simulink model "signal_tranmission"  (R2024b)
settings: Solver=ode45  StartTime=0.0  StopTime=10  FixedStep=0.000125  RelTol=1e-3
libraries: dspfdesign x500, commchan3 x1
(part 4 of 7)

== system signal_tranmission/SSB Modulator85 ==
  Input Signal : Inport
  Analog Filter Design : dspfdesign/Analog Filter Design  method=Butterworth  filttype=Bandpass  N=4  Wlo=438*2*pi  Whi=442*2*pi  Rp=2  Rs=40
  Balanced Modulator : Subsystem
  carrier signal : Sin  Frequency=440*2*pi  SampleTime=0
  Out1 : Outport
  wires:
  carrier signal/1 -> Balanced Modulator/2(Carrier Signal)
  Balanced Modulator/1(DSBSC) -> Analog Filter Design/1
  Analog Filter Design/1 -> Out1/1
  Input Signal/1 -> Balanced Modulator/1(Input Signal)

== system signal_tranmission/SSB Modulator86 ==
  Input Signal : Inport
  Analog Filter Design : dspfdesign/Analog Filter Design  method=Butterworth  filttype=Bandpass  N=4  Wlo=442*2*pi  Whi=446*2*pi  Rp=2  Rs=40
  Balanced Modulator : Subsystem
  carrier signal : Sin  Frequency=444*2*pi  SampleTime=0
  Out1 : Outport
  wires:
  carrier signal/1 -> Balanced Modulator/2(Carrier Signal)
  Balanced Modulator/1(DSBSC) -> Analog Filter Design/1
  Analog Filter Design/1 -> Out1/1
  Input Signal/1 -> Balanced Modulator/1(Input Signal)

== system signal_tranmission/SSB Modulator87 ==
  Input Signal : Inport
  Analog Filter Design : dspfdesign/Analog Filter Design  method=Butterworth  filttype=Bandpass  N=4  Wlo=446*2*pi  Whi=450*2*pi  Rp=2  Rs=40
  Balanced Modulator : Subsystem
  carrier signal : Sin  Frequency=448*2*pi  SampleTime=0
  Out1 : Outport
  wires:
  carrier signal/1 -> Balanced Modulator/2(Carrier Signal)
  Balanced Modulator/1(DSBSC) -> Analog Filter Design/1
  Analog Filter Design/1 -> Out1/1
  Input Signal/1 -> Balanced Modulator/1(Input Signal)

== system signal_tranmission/SSB Modulator88 ==
  Input Signal : Inport
  Analog Filter Design : dspfdesign/Analog Filter Design  method=Butterworth  filttype=Bandpass  N=4  Wlo=450*2*pi  Whi=454*2*pi  Rp=2  Rs=40
  Balanced Modulator : Subsystem
  carrier signal : Sin  Frequency=452*2*pi  SampleTime=0
  Out1 : Outport
  wires:
  carrier signal/1 -> Balanced Modulator/2(Carrier Signal)
  Balanced Modulator/1(DSBSC) -> Analog Filter Design/1
  Analog Filter Design/1 -> Out1/1
  Input Signal/1 -> Balanced Modulator/1(Input Signal)

== system signal_tranmission/SSB Modulator89 ==
  Input Signal : Inport
  Analog Filter Design : dspfdesign/Analog Filter Design  method=Butterworth  filttype=Bandpass  N=4  Wlo=454*2*pi  Whi=458*2*pi  Rp=2  Rs=40
  Balanced Modulator : Subsystem
  carrier signal : Sin  Frequency=456*2*pi  SampleTime=0
  Out1 : Outport
  wires:
  carrier signal/1 -> Balanced Modulator/2(Carrier Signal)
  Balanced Modulator/1(DSBSC) -> Analog Filter Design/1
  Analog Filter Design/1 -> Out1/1
  Input Signal/1 -> Balanced Modulator/1(Input Signal)

== system signal_tranmission/SSB Modulator9 ==
  Input Signal : Inport
  Analog Filter Design : dspfdesign/Analog Filter Design  method=Butterworth  filttype=Bandpass  N=4  Wlo=134*2*pi  Whi=138*2*pi  Rp=2  Rs=40
  Balanced Modulator : Subsystem
  carrier signal : Sin  Frequency=136*2*pi  SampleTime=0
  Out1 : Outport
  wires:
  carrier signal/1 -> Balanced Modulator/2(Carrier Signal)
  Balanced Modulator/1(DSBSC) -> Analog Filter Design/1
  Analog Filter Design/1 -> Out1/1
  Input Signal/1 -> Balanced Modulator/1(Input Signal)

== system signal_tranmission/SSB Modulator90 ==
  Input Signal : Inport
  Analog Filter Design : dspfdesign/Analog Filter Design  method=Butterworth  filttype=Bandpass  N=4  Wlo=458*2*pi  Whi=462*2*pi  Rp=2  Rs=40
  Balanced Modulator : Subsystem
  carrier signal : Sin  Frequency=460*2*pi  SampleTime=0
  Out1 : Outport
  wires:
  carrier signal/1 -> Balanced Modulator/2(Carrier Signal)
  Balanced Modulator/1(DSBSC) -> Analog Filter Design/1
  Analog Filter Design/1 -> Out1/1
  Input Signal/1 -> Balanced Modulator/1(Input Signal)

== system signal_tranmission/SSB Modulator91 ==
  Input Signal : Inport
  Analog Filter Design : dspfdesign/Analog Filter Design  method=Butterworth  filttype=Bandpass  N=4  Wlo=462*2*pi  Whi=466*2*pi  Rp=2  Rs=40
  Balanced Modulator : Subsystem
  carrier signal : Sin  Frequency=464*2*pi  SampleTime=0
  Out1 : Outport
  wires:
  carrier signal/1 -> Balanced Modulator/2(Carrier Signal)
  Balanced Modulator/1(DSBSC) -> Analog Filter Design/1
  Analog Filter Design/1 -> Out1/1
  Input Signal/1 -> Balanced Modulator/1(Input Signal)

== system signal_tranmission/SSB Modulator92 ==
  Input Signal : Inport
  Analog Filter Design : dspfdesign/Analog Filter Design  method=Butterworth  filttype=Bandpass  N=4  Wlo=466*2*pi  Whi=470*2*pi  Rp=2  Rs=40
  Balanced Modulator : Subsystem
  carrier signal : Sin  Frequency=468*2*pi  SampleTime=0
  Out1 : Outport
  wires:
  carrier signal/1 -> Balanced Modulator/2(Carrier Signal)
  Balanced Modulator/1(DSBSC) -> Analog Filter Design/1
  Analog Filter Design/1 -> Out1/1
  Input Signal/1 -> Balanced Modulator/1(Input Signal)

== system signal_tranmission/SSB Modulator93 ==
  Input Signal : Inport
  Analog Filter Design : dspfdesign/Analog Filter Design  method=Butterworth  filttype=Bandpass  N=4  Wlo=470*2*pi  Whi=474*2*pi  Rp=2  Rs=40
  Balanced Modulator : Subsystem
  carrier signal : Sin  Frequency=472*2*pi  SampleTime=0
  Out1 : Outport
  wires:
  carrier signal/1 -> Balanced Modulator/2(Carrier Signal)
  Balanced Modulator/1(DSBSC) -> Analog Filter Design/1
  Analog Filter Design/1 -> Out1/1
  Input Signal/1 -> Balanced Modulator/1(Input Signal)

== system signal_tranmission/SSB Modulator94 ==
  Input Signal : Inport
  Analog Filter Design : dspfdesign/Analog Filter Design  method=Butterworth  filttype=Bandpass  N=4  Wlo=474*2*pi  Whi=478*2*pi  Rp=2  Rs=40
  Balanced Modulator : Subsystem
  carrier signal : Sin  Frequency=476*2*pi  SampleTime=0
  Out1 : Outport
  wires:
  carrier signal/1 -> Balanced Modulator/2(Carrier Signal)
  Balanced Modulator/1(DSBSC) -> Analog Filter Design/1
  Analog Filter Design/1 -> Out1/1
  Input Signal/1 -> Balanced Modulator/1(Input Signal)

== system signal_tranmission/SSB Modulator95 ==
  Input Signal : Inport
  Analog Filter Design : dspfdesign/Analog Filter Design  method=Butterworth  filttype=Bandpass  N=4  Wlo=478*2*pi  Whi=482*2*pi  Rp=2  Rs=40
  Balanced Modulator : Subsystem
  carrier signal : Sin  Frequency=480*2*pi  SampleTime=0
  Out1 : Outport
  wires:
  carrier signal/1 -> Balanced Modulator/2(Carrier Signal)
  Balanced Modulator/1(DSBSC) -> Analog Filter Design/1
  Analog Filter Design/1 -> Out1/1
  Input Signal/1 -> Balanced Modulator/1(Input Signal)

== system signal_tranmission/SSB Modulator96 ==
  Input Signal : Inport
  Analog Filter Design : dspfdesign/Analog Filter Design  method=Butterworth  filttype=Bandpass  N=4  Wlo=482*2*pi  Whi=486*2*pi  Rp=2  Rs=40
  Balanced Modulator : Subsystem
  carrier signal : Sin  Frequency=484*2*pi  SampleTime=0
  Out1 : Outport
  wires:
  carrier signal/1 -> Balanced Modulator/2(Carrier Signal)
  Balanced Modulator/1(DSBSC) -> Analog Filter Design/1
  Analog Filter Design/1 -> Out1/1
  Input Signal/1 -> Balanced Modulator/1(Input Signal)

== system signal_tranmission/SSB Modulator97 ==
  Input Signal : Inport
  Analog Filter Design : dspfdesign/Analog Filter Design  method=Butterworth  filttype=Bandpass  N=4  Wlo=486*2*pi  Whi=490*2*pi  Rp=2  Rs=40
  Balanced Modulator : Subsystem
  carrier signal : Sin  Frequency=488*2*pi  SampleTime=0
  Out1 : Outport
  wires:
  carrier signal/1 -> Balanced Modulator/2(Carrier Signal)
  Balanced Modulator/1(DSBSC) -> Analog Filter Design/1
  Analog Filter Design/1 -> Out1/1
  Input Signal/1 -> Balanced Modulator/1(Input Signal)

== system signal_tranmission/SSB Modulator98 ==
  Input Signal : Inport
  Analog Filter Design : dspfdesign/Analog Filter Design  method=Butterworth  filttype=Bandpass  N=4  Wlo=490*2*pi  Whi=494*2*pi  Rp=2  Rs=40
  Balanced Modulator : Subsystem
  carrier signal : Sin  Frequency=492*2*pi  SampleTime=0
  Out1 : Outport
  wires:
  carrier signal/1 -> Balanced Modulator/2(Carrier Signal)
  Balanced Modulator/1(DSBSC) -> Analog Filter Design/1
  Analog Filter Design/1 -> Out1/1
  Input Signal/1 -> Balanced Modulator/1(Input Signal)

== system signal_tranmission/SSB Modulator99 ==
  Input Signal : Inport
  Analog Filter Design : dspfdesign/Analog Filter Design  method=Butterworth  filttype=Bandpass  N=4  Wlo=494*2*pi  Whi=498*2*pi  Rp=2  Rs=40
  Balanced Modulator : Subsystem
  carrier signal : Sin  Frequency=496*2*pi  SampleTime=0
  Out1 : Outport
  wires:
  carrier signal/1 -> Balanced Modulator/2(Carrier Signal)
  Balanced Modulator/1(DSBSC) -> Analog Filter Design/1
  Analog Filter Design/1 -> Out1/1
  Input Signal/1 -> Balanced Modulator/1(Input Signal)

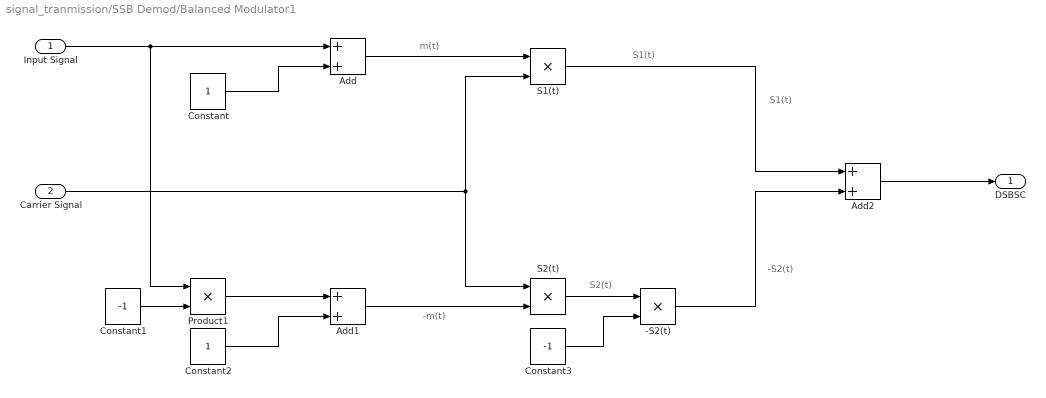
== system signal_tranmission/SSB Demod/Balanced Modulator1 ==
  note: -S2(t)
  note: S1(t)
  note: -m(t)
  note: m(t)
  note: S2(t)
  note: S1(t)
  Input Signal : Inport
  Carrier Signal : Inport  Port=2
  -S2(t) : Product
  Add : Sum
  Add1 : Sum
  Add2 : Sum
  Constant : Constant
  Constant1 : Constant  Value=-1
  Constant2 : Constant
  Constant3 : Constant  Value=-1
  Product1 : Product
  S1(t) : Product
  S2(t) : Product
  DSBSC : Outport
  wires:
  Product1/1 -> Add1/1
  Add/1 -> S1(t)/1
  Constant3/1 -> -S2(t)/2
  Constant2/1 -> Add1/2
  S2(t)/1 -> -S2(t)/1
  Carrier Signal/1 -> S1(t)/2, S2(t)/1
  Constant/1 -> Add/2
  Add1/1 -> S2(t)/2
  Constant1/1 -> Product1/2
  -S2(t)/1 -> Add2/2
  S1(t)/1 -> Add2/1
  Input Signal/1 -> Product1/1, Add/1
  Add2/1 -> DSBSC/1

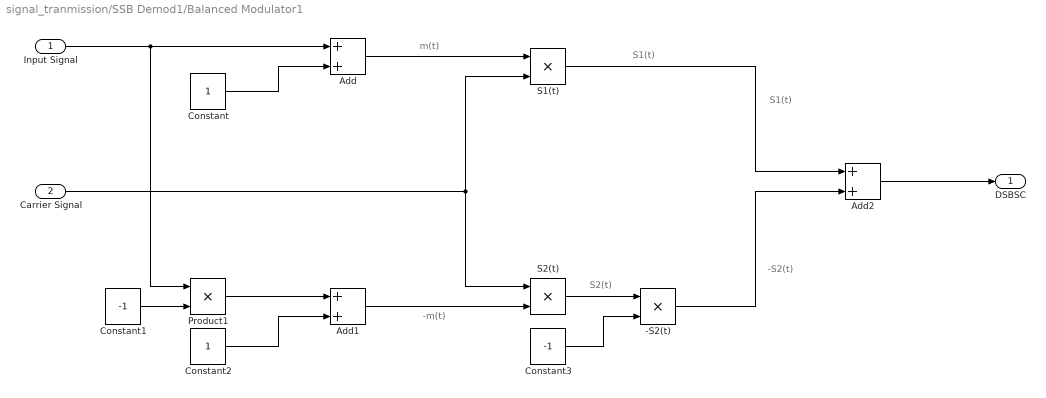
== system signal_tranmission/SSB Demod1/Balanced Modulator1 ==
  note: -S2(t)
  note: S1(t)
  note: -m(t)
  note: m(t)
  note: S2(t)
  note: S1(t)
  Input Signal : Inport
  Carrier Signal : Inport  Port=2
  -S2(t) : Product
  Add : Sum
  Add1 : Sum
  Add2 : Sum
  Constant : Constant
  Constant1 : Constant  Value=-1
  Constant2 : Constant
  Constant3 : Constant  Value=-1
  Product1 : Product
  S1(t) : Product
  S2(t) : Product
  DSBSC : Outport
  wires:
  Product1/1 -> Add1/1
  Add/1 -> S1(t)/1
  Constant3/1 -> -S2(t)/2
  Constant2/1 -> Add1/2
  S2(t)/1 -> -S2(t)/1
  Carrier Signal/1 -> S1(t)/2, S2(t)/1
  Constant/1 -> Add/2
  Add1/1 -> S2(t)/2
  Constant1/1 -> Product1/2
  -S2(t)/1 -> Add2/2
  S1(t)/1 -> Add2/1
  Input Signal/1 -> Product1/1, Add/1
  Add2/1 -> DSBSC/1

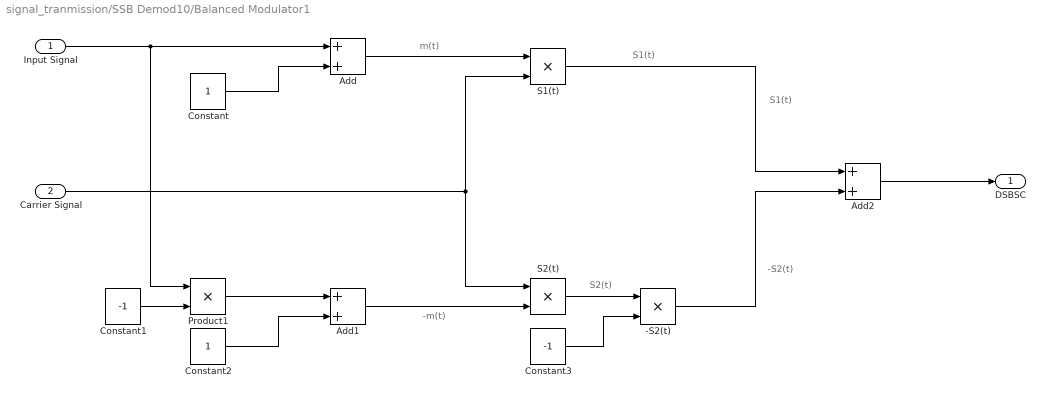
== system signal_tranmission/SSB Demod10/Balanced Modulator1 ==
  note: -S2(t)
  note: S1(t)
  note: -m(t)
  note: m(t)
  note: S2(t)
  note: S1(t)
  Input Signal : Inport
  Carrier Signal : Inport  Port=2
  -S2(t) : Product
  Add : Sum
  Add1 : Sum
  Add2 : Sum
  Constant : Constant
  Constant1 : Constant  Value=-1
  Constant2 : Constant
  Constant3 : Constant  Value=-1
  Product1 : Product
  S1(t) : Product
  S2(t) : Product
  DSBSC : Outport
  wires:
  Product1/1 -> Add1/1
  Add/1 -> S1(t)/1
  Constant3/1 -> -S2(t)/2
  Constant2/1 -> Add1/2
  S2(t)/1 -> -S2(t)/1
  Carrier Signal/1 -> S1(t)/2, S2(t)/1
  Constant/1 -> Add/2
  Add1/1 -> S2(t)/2
  Constant1/1 -> Product1/2
  -S2(t)/1 -> Add2/2
  S1(t)/1 -> Add2/1
  Input Signal/1 -> Product1/1, Add/1
  Add2/1 -> DSBSC/1

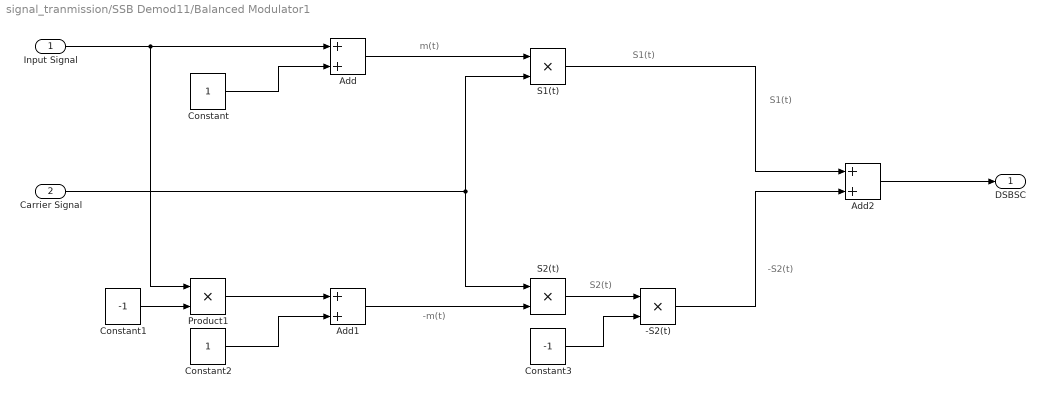
== system signal_tranmission/SSB Demod11/Balanced Modulator1 ==
  note: -S2(t)
  note: S1(t)
  note: -m(t)
  note: m(t)
  note: S2(t)
  note: S1(t)
  Input Signal : Inport
  Carrier Signal : Inport  Port=2
  -S2(t) : Product
  Add : Sum
  Add1 : Sum
  Add2 : Sum
  Constant : Constant
  Constant1 : Constant  Value=-1
  Constant2 : Constant
  Constant3 : Constant  Value=-1
  Product1 : Product
  S1(t) : Product
  S2(t) : Product
  DSBSC : Outport
  wires:
  Product1/1 -> Add1/1
  Add/1 -> S1(t)/1
  Constant3/1 -> -S2(t)/2
  Constant2/1 -> Add1/2
  S2(t)/1 -> -S2(t)/1
  Carrier Signal/1 -> S1(t)/2, S2(t)/1
  Constant/1 -> Add/2
  Add1/1 -> S2(t)/2
  Constant1/1 -> Product1/2
  -S2(t)/1 -> Add2/2
  S1(t)/1 -> Add2/1
  Input Signal/1 -> Product1/1, Add/1
  Add2/1 -> DSBSC/1

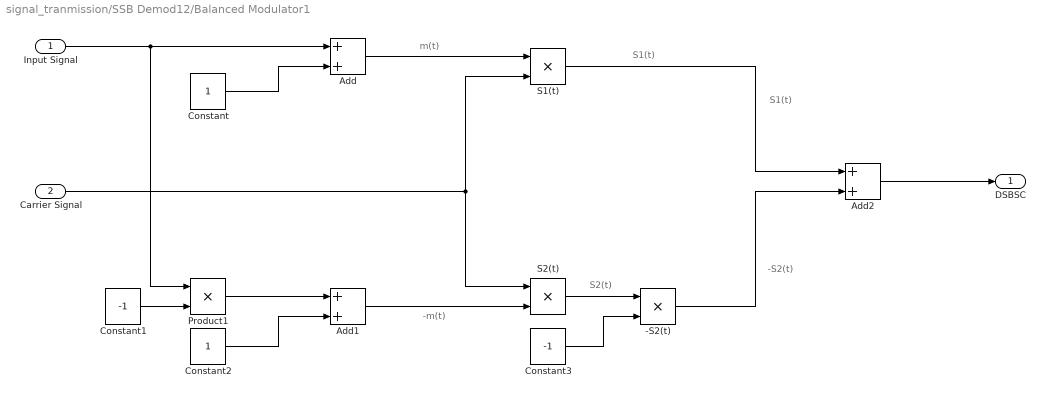
== system signal_tranmission/SSB Demod12/Balanced Modulator1 ==
  note: -S2(t)
  note: S1(t)
  note: -m(t)
  note: m(t)
  note: S2(t)
  note: S1(t)
  Input Signal : Inport
  Carrier Signal : Inport  Port=2
  -S2(t) : Product
  Add : Sum
  Add1 : Sum
  Add2 : Sum
  Constant : Constant
  Constant1 : Constant  Value=-1
  Constant2 : Constant
  Constant3 : Constant  Value=-1
  Product1 : Product
  S1(t) : Product
  S2(t) : Product
  DSBSC : Outport
  wires:
  Product1/1 -> Add1/1
  Add/1 -> S1(t)/1
  Constant3/1 -> -S2(t)/2
  Constant2/1 -> Add1/2
  S2(t)/1 -> -S2(t)/1
  Carrier Signal/1 -> S1(t)/2, S2(t)/1
  Constant/1 -> Add/2
  Add1/1 -> S2(t)/2
  Constant1/1 -> Product1/2
  -S2(t)/1 -> Add2/2
  S1(t)/1 -> Add2/1
  Input Signal/1 -> Product1/1, Add/1
  Add2/1 -> DSBSC/1

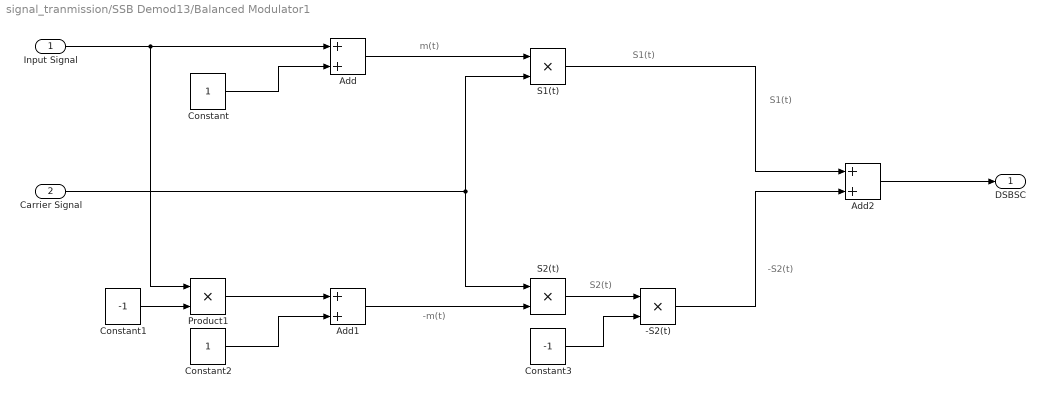
== system signal_tranmission/SSB Demod13/Balanced Modulator1 ==
  note: -S2(t)
  note: S1(t)
  note: -m(t)
  note: m(t)
  note: S2(t)
  note: S1(t)
  Input Signal : Inport
  Carrier Signal : Inport  Port=2
  -S2(t) : Product
  Add : Sum
  Add1 : Sum
  Add2 : Sum
  Constant : Constant
  Constant1 : Constant  Value=-1
  Constant2 : Constant
  Constant3 : Constant  Value=-1
  Product1 : Product
  S1(t) : Product
  S2(t) : Product
  DSBSC : Outport
  wires:
  Product1/1 -> Add1/1
  Add/1 -> S1(t)/1
  Constant3/1 -> -S2(t)/2
  Constant2/1 -> Add1/2
  S2(t)/1 -> -S2(t)/1
  Carrier Signal/1 -> S1(t)/2, S2(t)/1
  Constant/1 -> Add/2
  Add1/1 -> S2(t)/2
  Constant1/1 -> Product1/2
  -S2(t)/1 -> Add2/2
  S1(t)/1 -> Add2/1
  Input Signal/1 -> Product1/1, Add/1
  Add2/1 -> DSBSC/1

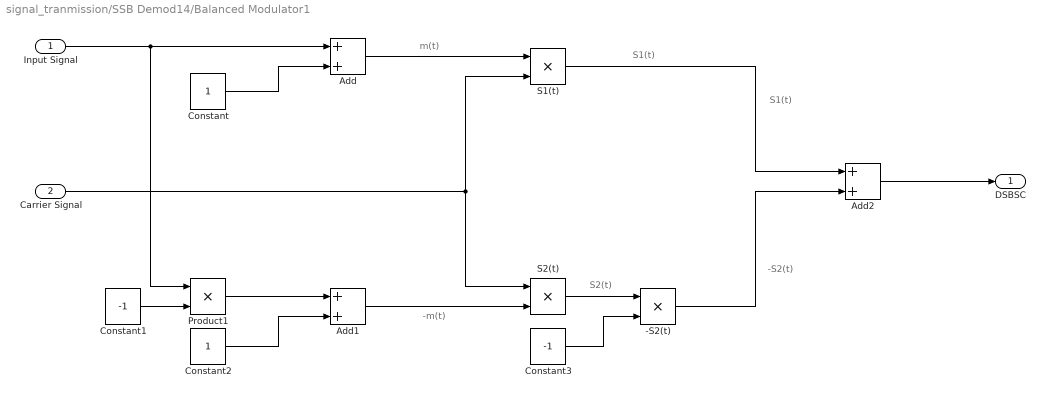
== system signal_tranmission/SSB Demod14/Balanced Modulator1 ==
  note: -S2(t)
  note: S1(t)
  note: -m(t)
  note: m(t)
  note: S2(t)
  note: S1(t)
  Input Signal : Inport
  Carrier Signal : Inport  Port=2
  -S2(t) : Product
  Add : Sum
  Add1 : Sum
  Add2 : Sum
  Constant : Constant
  Constant1 : Constant  Value=-1
  Constant2 : Constant
  Constant3 : Constant  Value=-1
  Product1 : Product
  S1(t) : Product
  S2(t) : Product
  DSBSC : Outport
  wires:
  Product1/1 -> Add1/1
  Add/1 -> S1(t)/1
  Constant3/1 -> -S2(t)/2
  Constant2/1 -> Add1/2
  S2(t)/1 -> -S2(t)/1
  Carrier Signal/1 -> S1(t)/2, S2(t)/1
  Constant/1 -> Add/2
  Add1/1 -> S2(t)/2
  Constant1/1 -> Product1/2
  -S2(t)/1 -> Add2/2
  S1(t)/1 -> Add2/1
  Input Signal/1 -> Product1/1, Add/1
  Add2/1 -> DSBSC/1

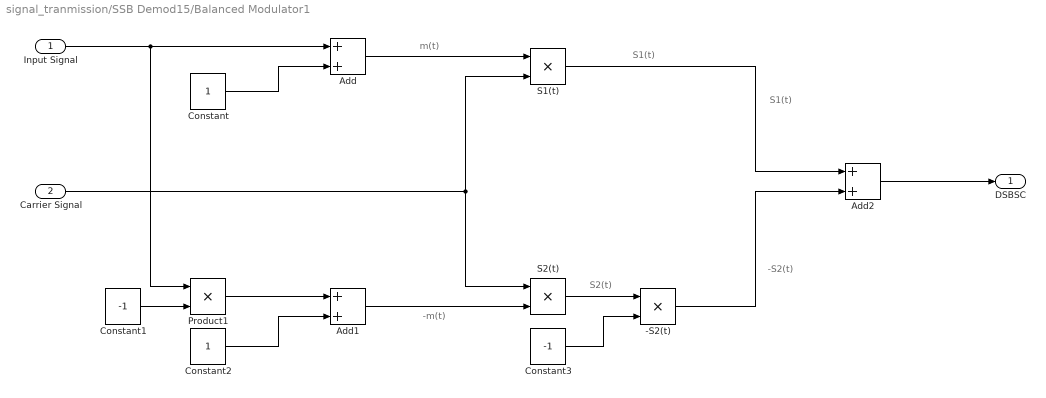
== system signal_tranmission/SSB Demod15/Balanced Modulator1 ==
  note: -S2(t)
  note: S1(t)
  note: -m(t)
  note: m(t)
  note: S2(t)
  note: S1(t)
  Input Signal : Inport
  Carrier Signal : Inport  Port=2
  -S2(t) : Product
  Add : Sum
  Add1 : Sum
  Add2 : Sum
  Constant : Constant
  Constant1 : Constant  Value=-1
  Constant2 : Constant
  Constant3 : Constant  Value=-1
  Product1 : Product
  S1(t) : Product
  S2(t) : Product
  DSBSC : Outport
  wires:
  Product1/1 -> Add1/1
  Add/1 -> S1(t)/1
  Constant3/1 -> -S2(t)/2
  Constant2/1 -> Add1/2
  S2(t)/1 -> -S2(t)/1
  Carrier Signal/1 -> S1(t)/2, S2(t)/1
  Constant/1 -> Add/2
  Add1/1 -> S2(t)/2
  Constant1/1 -> Product1/2
  -S2(t)/1 -> Add2/2
  S1(t)/1 -> Add2/1
  Input Signal/1 -> Product1/1, Add/1
  Add2/1 -> DSBSC/1

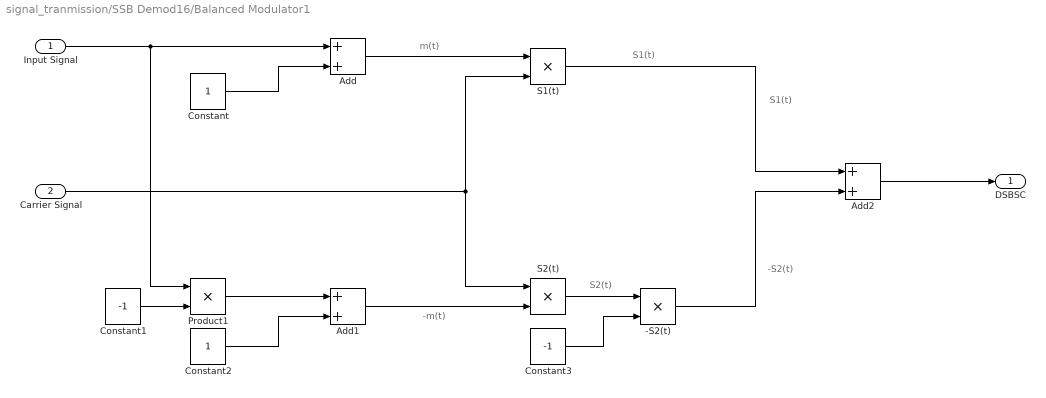
== system signal_tranmission/SSB Demod16/Balanced Modulator1 ==
  note: -S2(t)
  note: S1(t)
  note: -m(t)
  note: m(t)
  note: S2(t)
  note: S1(t)
  Input Signal : Inport
  Carrier Signal : Inport  Port=2
  -S2(t) : Product
  Add : Sum
  Add1 : Sum
  Add2 : Sum
  Constant : Constant
  Constant1 : Constant  Value=-1
  Constant2 : Constant
  Constant3 : Constant  Value=-1
  Product1 : Product
  S1(t) : Product
  S2(t) : Product
  DSBSC : Outport
  wires:
  Product1/1 -> Add1/1
  Add/1 -> S1(t)/1
  Constant3/1 -> -S2(t)/2
  Constant2/1 -> Add1/2
  S2(t)/1 -> -S2(t)/1
  Carrier Signal/1 -> S1(t)/2, S2(t)/1
  Constant/1 -> Add/2
  Add1/1 -> S2(t)/2
  Constant1/1 -> Product1/2
  -S2(t)/1 -> Add2/2
  S1(t)/1 -> Add2/1
  Input Signal/1 -> Product1/1, Add/1
  Add2/1 -> DSBSC/1

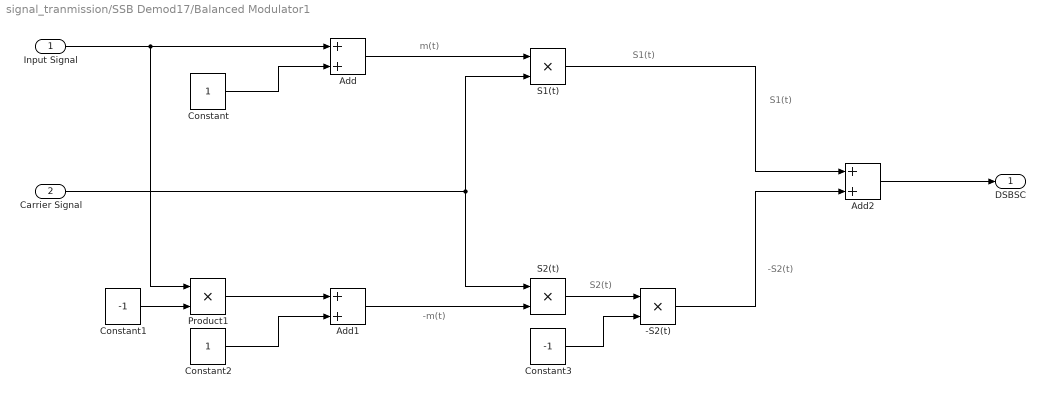
== system signal_tranmission/SSB Demod17/Balanced Modulator1 ==
  note: -S2(t)
  note: S1(t)
  note: -m(t)
  note: m(t)
  note: S2(t)
  note: S1(t)
  Input Signal : Inport
  Carrier Signal : Inport  Port=2
  -S2(t) : Product
  Add : Sum
  Add1 : Sum
  Add2 : Sum
  Constant : Constant
  Constant1 : Constant  Value=-1
  Constant2 : Constant
  Constant3 : Constant  Value=-1
  Product1 : Product
  S1(t) : Product
  S2(t) : Product
  DSBSC : Outport
  wires:
  Product1/1 -> Add1/1
  Add/1 -> S1(t)/1
  Constant3/1 -> -S2(t)/2
  Constant2/1 -> Add1/2
  S2(t)/1 -> -S2(t)/1
  Carrier Signal/1 -> S1(t)/2, S2(t)/1
  Constant/1 -> Add/2
  Add1/1 -> S2(t)/2
  Constant1/1 -> Product1/2
  -S2(t)/1 -> Add2/2
  S1(t)/1 -> Add2/1
  Input Signal/1 -> Product1/1, Add/1
  Add2/1 -> DSBSC/1

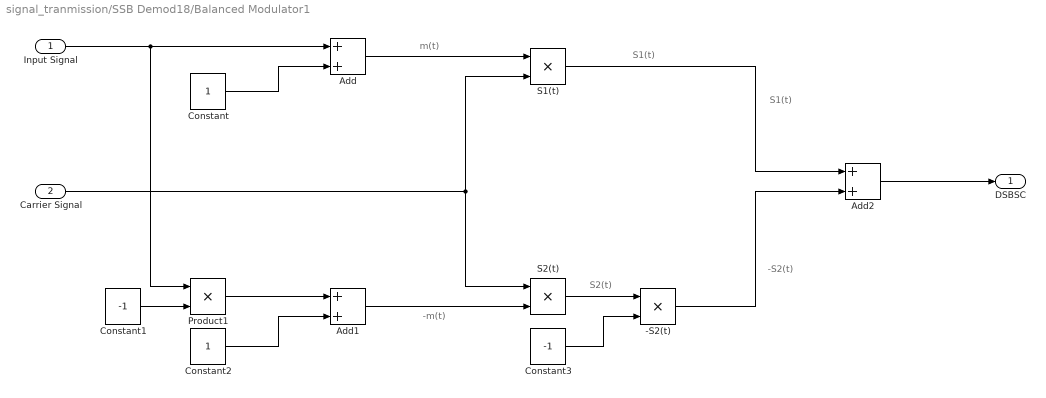
== system signal_tranmission/SSB Demod18/Balanced Modulator1 ==
  note: -S2(t)
  note: S1(t)
  note: -m(t)
  note: m(t)
  note: S2(t)
  note: S1(t)
  Input Signal : Inport
  Carrier Signal : Inport  Port=2
  -S2(t) : Product
  Add : Sum
  Add1 : Sum
  Add2 : Sum
  Constant : Constant
  Constant1 : Constant  Value=-1
  Constant2 : Constant
  Constant3 : Constant  Value=-1
  Product1 : Product
  S1(t) : Product
  S2(t) : Product
  DSBSC : Outport
  wires:
  Product1/1 -> Add1/1
  Add/1 -> S1(t)/1
  Constant3/1 -> -S2(t)/2
  Constant2/1 -> Add1/2
  S2(t)/1 -> -S2(t)/1
  Carrier Signal/1 -> S1(t)/2, S2(t)/1
  Constant/1 -> Add/2
  Add1/1 -> S2(t)/2
  Constant1/1 -> Product1/2
  -S2(t)/1 -> Add2/2
  S1(t)/1 -> Add2/1
  Input Signal/1 -> Product1/1, Add/1
  Add2/1 -> DSBSC/1

== system signal_tranmission/SSB Demod19/Balanced Modulator1 ==
  note: -S2(t)
  note: S1(t)
  note: -m(t)
  note: m(t)
  note: S2(t)
  note: S1(t)
  Input Signal : Inport
  Carrier Signal : Inport  Port=2
  -S2(t) : Product
  Add : Sum
  Add1 : Sum
  Add2 : Sum
  Constant : Constant
  Constant1 : Constant  Value=-1
  Constant2 : Constant
  Constant3 : Constant  Value=-1
  Product1 : Product
  S1(t) : Product
  S2(t) : Product
  DSBSC : Outport
  wires:
  Product1/1 -> Add1/1
  Add/1 -> S1(t)/1
  Constant3/1 -> -S2(t)/2
  Constant2/1 -> Add1/2
  S2(t)/1 -> -S2(t)/1
  Carrier Signal/1 -> S1(t)/2, S2(t)/1
  Constant/1 -> Add/2
  Add1/1 -> S2(t)/2
  Constant1/1 -> Product1/2
  -S2(t)/1 -> Add2/2
  S1(t)/1 -> Add2/1
  Input Signal/1 -> Product1/1, Add/1
  Add2/1 -> DSBSC/1

== system signal_tranmission/SSB Demod2/Balanced Modulator1 ==
  note: -S2(t)
  note: S1(t)
  note: -m(t)
  note: m(t)
  note: S2(t)
  note: S1(t)
  Input Signal : Inport
  Carrier Signal : Inport  Port=2
  -S2(t) : Product
  Add : Sum
  Add1 : Sum
  Add2 : Sum
  Constant : Constant
  Constant1 : Constant  Value=-1
  Constant2 : Constant
  Constant3 : Constant  Value=-1
  Product1 : Product
  S1(t) : Product
  S2(t) : Product
  DSBSC : Outport
  wires:
  Product1/1 -> Add1/1
  Add/1 -> S1(t)/1
  Constant3/1 -> -S2(t)/2
  Constant2/1 -> Add1/2
  S2(t)/1 -> -S2(t)/1
  Carrier Signal/1 -> S1(t)/2, S2(t)/1
  Constant/1 -> Add/2
  Add1/1 -> S2(t)/2
  Constant1/1 -> Product1/2
  -S2(t)/1 -> Add2/2
  S1(t)/1 -> Add2/1
  Input Signal/1 -> Product1/1, Add/1
  Add2/1 -> DSBSC/1

== system signal_tranmission/SSB Demod20/Balanced Modulator1 ==
  note: -S2(t)
  note: S1(t)
  note: -m(t)
  note: m(t)
  note: S2(t)
  note: S1(t)
  Input Signal : Inport
  Carrier Signal : Inport  Port=2
  -S2(t) : Product
  Add : Sum
  Add1 : Sum
  Add2 : Sum
  Constant : Constant
  Constant1 : Constant  Value=-1
  Constant2 : Constant
  Constant3 : Constant  Value=-1
  Product1 : Product
  S1(t) : Product
  S2(t) : Product
  DSBSC : Outport
  wires:
  Product1/1 -> Add1/1
  Add/1 -> S1(t)/1
  Constant3/1 -> -S2(t)/2
  Constant2/1 -> Add1/2
  S2(t)/1 -> -S2(t)/1
  Carrier Signal/1 -> S1(t)/2, S2(t)/1
  Constant/1 -> Add/2
  Add1/1 -> S2(t)/2
  Constant1/1 -> Product1/2
  -S2(t)/1 -> Add2/2
  S1(t)/1 -> Add2/1
  Input Signal/1 -> Product1/1, Add/1
  Add2/1 -> DSBSC/1

== system signal_tranmission/SSB Demod21/Balanced Modulator1 ==
  note: -S2(t)
  note: S1(t)
  note: -m(t)
  note: m(t)
  note: S2(t)
  note: S1(t)
  Input Signal : Inport
  Carrier Signal : Inport  Port=2
  -S2(t) : Product
  Add : Sum
  Add1 : Sum
  Add2 : Sum
  Constant : Constant
  Constant1 : Constant  Value=-1
  Constant2 : Constant
  Constant3 : Constant  Value=-1
  Product1 : Product
  S1(t) : Product
  S2(t) : Product
  DSBSC : Outport
  wires:
  Product1/1 -> Add1/1
  Add/1 -> S1(t)/1
  Constant3/1 -> -S2(t)/2
  Constant2/1 -> Add1/2
  S2(t)/1 -> -S2(t)/1
  Carrier Signal/1 -> S1(t)/2, S2(t)/1
  Constant/1 -> Add/2
  Add1/1 -> S2(t)/2
  Constant1/1 -> Product1/2
  -S2(t)/1 -> Add2/2
  S1(t)/1 -> Add2/1
  Input Signal/1 -> Product1/1, Add/1
  Add2/1 -> DSBSC/1

== system signal_tranmission/SSB Demod22/Balanced Modulator1 ==
  note: -S2(t)
  note: S1(t)
  note: -m(t)
  note: m(t)
  note: S2(t)
  note: S1(t)
  Input Signal : Inport
  Carrier Signal : Inport  Port=2
  -S2(t) : Product
  Add : Sum
  Add1 : Sum
  Add2 : Sum
  Constant : Constant
  Constant1 : Constant  Value=-1
  Constant2 : Constant
  Constant3 : Constant  Value=-1
  Product1 : Product
  S1(t) : Product
  S2(t) : Product
  DSBSC : Outport
  wires:
  Product1/1 -> Add1/1
  Add/1 -> S1(t)/1
  Constant3/1 -> -S2(t)/2
  Constant2/1 -> Add1/2
  S2(t)/1 -> -S2(t)/1
  Carrier Signal/1 -> S1(t)/2, S2(t)/1
  Constant/1 -> Add/2
  Add1/1 -> S2(t)/2
  Constant1/1 -> Product1/2
  -S2(t)/1 -> Add2/2
  S1(t)/1 -> Add2/1
  Input Signal/1 -> Product1/1, Add/1
  Add2/1 -> DSBSC/1

== system signal_tranmission/SSB Demod23/Balanced Modulator1 ==
  note: -S2(t)
  note: S1(t)
  note: -m(t)
  note: m(t)
  note: S2(t)
  note: S1(t)
  Input Signal : Inport
  Carrier Signal : Inport  Port=2
  -S2(t) : Product
  Add : Sum
  Add1 : Sum
  Add2 : Sum
  Constant : Constant
  Constant1 : Constant  Value=-1
  Constant2 : Constant
  Constant3 : Constant  Value=-1
  Product1 : Product
  S1(t) : Product
  S2(t) : Product
  DSBSC : Outport
  wires:
  Product1/1 -> Add1/1
  Add/1 -> S1(t)/1
  Constant3/1 -> -S2(t)/2
  Constant2/1 -> Add1/2
  S2(t)/1 -> -S2(t)/1
  Carrier Signal/1 -> S1(t)/2, S2(t)/1
  Constant/1 -> Add/2
  Add1/1 -> S2(t)/2
  Constant1/1 -> Product1/2
  -S2(t)/1 -> Add2/2
  S1(t)/1 -> Add2/1
  Input Signal/1 -> Product1/1, Add/1
  Add2/1 -> DSBSC/1

== system signal_tranmission/SSB Demod24/Balanced Modulator1 ==
  note: -S2(t)
  note: S1(t)
  note: -m(t)
  note: m(t)
  note: S2(t)
  note: S1(t)
  Input Signal : Inport
  Carrier Signal : Inport  Port=2
  -S2(t) : Product
  Add : Sum
  Add1 : Sum
  Add2 : Sum
  Constant : Constant
  Constant1 : Constant  Value=-1
  Constant2 : Constant
  Constant3 : Constant  Value=-1
  Product1 : Product
  S1(t) : Product
  S2(t) : Product
  DSBSC : Outport
  wires:
  Product1/1 -> Add1/1
  Add/1 -> S1(t)/1
  Constant3/1 -> -S2(t)/2
  Constant2/1 -> Add1/2
  S2(t)/1 -> -S2(t)/1
  Carrier Signal/1 -> S1(t)/2, S2(t)/1
  Constant/1 -> Add/2
  Add1/1 -> S2(t)/2
  Constant1/1 -> Product1/2
  -S2(t)/1 -> Add2/2
  S1(t)/1 -> Add2/1
  Input Signal/1 -> Product1/1, Add/1
  Add2/1 -> DSBSC/1

== system signal_tranmission/SSB Demod25/Balanced Modulator1 ==
  note: -S2(t)
  note: S1(t)
  note: -m(t)
  note: m(t)
  note: S2(t)
  note: S1(t)
  Input Signal : Inport
  Carrier Signal : Inport  Port=2
  -S2(t) : Product
  Add : Sum
  Add1 : Sum
  Add2 : Sum
  Constant : Constant
  Constant1 : Constant  Value=-1
  Constant2 : Constant
  Constant3 : Constant  Value=-1
  Product1 : Product
  S1(t) : Product
  S2(t) : Product
  DSBSC : Outport
  wires:
  Product1/1 -> Add1/1
  Add/1 -> S1(t)/1
  Constant3/1 -> -S2(t)/2
  Constant2/1 -> Add1/2
  S2(t)/1 -> -S2(t)/1
  Carrier Signal/1 -> S1(t)/2, S2(t)/1
  Constant/1 -> Add/2
  Add1/1 -> S2(t)/2
  Constant1/1 -> Product1/2
  -S2(t)/1 -> Add2/2
  S1(t)/1 -> Add2/1
  Input Signal/1 -> Product1/1, Add/1
  Add2/1 -> DSBSC/1

== system signal_tranmission/SSB Demod26/Balanced Modulator1 ==
  note: -S2(t)
  note: S1(t)
  note: -m(t)
  note: m(t)
  note: S2(t)
  note: S1(t)
  Input Signal : Inport
  Carrier Signal : Inport  Port=2
  -S2(t) : Product
  Add : Sum
  Add1 : Sum
  Add2 : Sum
  Constant : Constant
  Constant1 : Constant  Value=-1
  Constant2 : Constant
  Constant3 : Constant  Value=-1
  Product1 : Product
  S1(t) : Product
  S2(t) : Product
  DSBSC : Outport
  wires:
  Product1/1 -> Add1/1
  Add/1 -> S1(t)/1
  Constant3/1 -> -S2(t)/2
  Constant2/1 -> Add1/2
  S2(t)/1 -> -S2(t)/1
  Carrier Signal/1 -> S1(t)/2, S2(t)/1
  Constant/1 -> Add/2
  Add1/1 -> S2(t)/2
  Constant1/1 -> Product1/2
  -S2(t)/1 -> Add2/2
  S1(t)/1 -> Add2/1
  Input Signal/1 -> Product1/1, Add/1
  Add2/1 -> DSBSC/1

== system signal_tranmission/SSB Demod27/Balanced Modulator1 ==
  note: -S2(t)
  note: S1(t)
  note: -m(t)
  note: m(t)
  note: S2(t)
  note: S1(t)
  Input Signal : Inport
  Carrier Signal : Inport  Port=2
  -S2(t) : Product
  Add : Sum
  Add1 : Sum
  Add2 : Sum
  Constant : Constant
  Constant1 : Constant  Value=-1
  Constant2 : Constant
  Constant3 : Constant  Value=-1
  Product1 : Product
  S1(t) : Product
  S2(t) : Product
  DSBSC : Outport
  wires:
  Product1/1 -> Add1/1
  Add/1 -> S1(t)/1
  Constant3/1 -> -S2(t)/2
  Constant2/1 -> Add1/2
  S2(t)/1 -> -S2(t)/1
  Carrier Signal/1 -> S1(t)/2, S2(t)/1
  Constant/1 -> Add/2
  Add1/1 -> S2(t)/2
  Constant1/1 -> Product1/2
  -S2(t)/1 -> Add2/2
  S1(t)/1 -> Add2/1
  Input Signal/1 -> Product1/1, Add/1
  Add2/1 -> DSBSC/1

== system signal_tranmission/SSB Demod28/Balanced Modulator1 ==
  note: -S2(t)
  note: S1(t)
  note: -m(t)
  note: m(t)
  note: S2(t)
  note: S1(t)
  Input Signal : Inport
  Carrier Signal : Inport  Port=2
  -S2(t) : Product
  Add : Sum
  Add1 : Sum
  Add2 : Sum
  Constant : Constant
  Constant1 : Constant  Value=-1
  Constant2 : Constant
  Constant3 : Constant  Value=-1
  Product1 : Product
  S1(t) : Product
  S2(t) : Product
  DSBSC : Outport
  wires:
  Product1/1 -> Add1/1
  Add/1 -> S1(t)/1
  Constant3/1 -> -S2(t)/2
  Constant2/1 -> Add1/2
  S2(t)/1 -> -S2(t)/1
  Carrier Signal/1 -> S1(t)/2, S2(t)/1
  Constant/1 -> Add/2
  Add1/1 -> S2(t)/2
  Constant1/1 -> Product1/2
  -S2(t)/1 -> Add2/2
  S1(t)/1 -> Add2/1
  Input Signal/1 -> Product1/1, Add/1
  Add2/1 -> DSBSC/1

== system signal_tranmission/SSB Demod29/Balanced Modulator1 ==
  note: -S2(t)
  note: S1(t)
  note: -m(t)
  note: m(t)
  note: S2(t)
  note: S1(t)
  Input Signal : Inport
  Carrier Signal : Inport  Port=2
  -S2(t) : Product
  Add : Sum
  Add1 : Sum
  Add2 : Sum
  Constant : Constant
  Constant1 : Constant  Value=-1
  Constant2 : Constant
  Constant3 : Constant  Value=-1
  Product1 : Product
  S1(t) : Product
  S2(t) : Product
  DSBSC : Outport
  wires:
  Product1/1 -> Add1/1
  Add/1 -> S1(t)/1
  Constant3/1 -> -S2(t)/2
  Constant2/1 -> Add1/2
  S2(t)/1 -> -S2(t)/1
  Carrier Signal/1 -> S1(t)/2, S2(t)/1
  Constant/1 -> Add/2
  Add1/1 -> S2(t)/2
  Constant1/1 -> Product1/2
  -S2(t)/1 -> Add2/2
  S1(t)/1 -> Add2/1
  Input Signal/1 -> Product1/1, Add/1
  Add2/1 -> DSBSC/1

== system signal_tranmission/SSB Demod3/Balanced Modulator1 ==
  note: -S2(t)
  note: S1(t)
  note: -m(t)
  note: m(t)
  note: S2(t)
  note: S1(t)
  Input Signal : Inport
  Carrier Signal : Inport  Port=2
  -S2(t) : Product
  Add : Sum
  Add1 : Sum
  Add2 : Sum
  Constant : Constant
  Constant1 : Constant  Value=-1
  Constant2 : Constant
  Constant3 : Constant  Value=-1
  Product1 : Product
  S1(t) : Product
  S2(t) : Product
  DSBSC : Outport
  wires:
  Product1/1 -> Add1/1
  Add/1 -> S1(t)/1
  Constant3/1 -> -S2(t)/2
  Constant2/1 -> Add1/2
  S2(t)/1 -> -S2(t)/1
  Carrier Signal/1 -> S1(t)/2, S2(t)/1
  Constant/1 -> Add/2
  Add1/1 -> S2(t)/2
  Constant1/1 -> Product1/2
  -S2(t)/1 -> Add2/2
  S1(t)/1 -> Add2/1
  Input Signal/1 -> Product1/1, Add/1
  Add2/1 -> DSBSC/1

== system signal_tranmission/SSB Demod30/Balanced Modulator1 ==
  note: -S2(t)
  note: S1(t)
  note: -m(t)
  note: m(t)
  note: S2(t)
  note: S1(t)
  Input Signal : Inport
  Carrier Signal : Inport  Port=2
  -S2(t) : Product
  Add : Sum
  Add1 : Sum
  Add2 : Sum
  Constant : Constant
  Constant1 : Constant  Value=-1
  Constant2 : Constant
  Constant3 : Constant  Value=-1
  Product1 : Product
  S1(t) : Product
  S2(t) : Product
  DSBSC : Outport
  wires:
  Product1/1 -> Add1/1
  Add/1 -> S1(t)/1
  Constant3/1 -> -S2(t)/2
  Constant2/1 -> Add1/2
  S2(t)/1 -> -S2(t)/1
  Carrier Signal/1 -> S1(t)/2, S2(t)/1
  Constant/1 -> Add/2
  Add1/1 -> S2(t)/2
  Constant1/1 -> Product1/2
  -S2(t)/1 -> Add2/2
  S1(t)/1 -> Add2/1
  Input Signal/1 -> Product1/1, Add/1
  Add2/1 -> DSBSC/1

== system signal_tranmission/SSB Demod31/Balanced Modulator1 ==
  note: -S2(t)
  note: S1(t)
  note: -m(t)
  note: m(t)
  note: S2(t)
  note: S1(t)
  Input Signal : Inport
  Carrier Signal : Inport  Port=2
  -S2(t) : Product
  Add : Sum
  Add1 : Sum
  Add2 : Sum
  Constant : Constant
  Constant1 : Constant  Value=-1
  Constant2 : Constant
  Constant3 : Constant  Value=-1
  Product1 : Product
  S1(t) : Product
  S2(t) : Product
  DSBSC : Outport
  wires:
  Product1/1 -> Add1/1
  Add/1 -> S1(t)/1
  Constant3/1 -> -S2(t)/2
  Constant2/1 -> Add1/2
  S2(t)/1 -> -S2(t)/1
  Carrier Signal/1 -> S1(t)/2, S2(t)/1
  Constant/1 -> Add/2
  Add1/1 -> S2(t)/2
  Constant1/1 -> Product1/2
  -S2(t)/1 -> Add2/2
  S1(t)/1 -> Add2/1
  Input Signal/1 -> Product1/1, Add/1
  Add2/1 -> DSBSC/1

== system signal_tranmission/SSB Demod32/Balanced Modulator1 ==
  note: -S2(t)
  note: S1(t)
  note: -m(t)
  note: m(t)
  note: S2(t)
  note: S1(t)
  Input Signal : Inport
  Carrier Signal : Inport  Port=2
  -S2(t) : Product
  Add : Sum
  Add1 : Sum
  Add2 : Sum
  Constant : Constant
  Constant1 : Constant  Value=-1
  Constant2 : Constant
  Constant3 : Constant  Value=-1
  Product1 : Product
  S1(t) : Product
  S2(t) : Product
  DSBSC : Outport
  wires:
  Product1/1 -> Add1/1
  Add/1 -> S1(t)/1
  Constant3/1 -> -S2(t)/2
  Constant2/1 -> Add1/2
  S2(t)/1 -> -S2(t)/1
  Carrier Signal/1 -> S1(t)/2, S2(t)/1
  Constant/1 -> Add/2
  Add1/1 -> S2(t)/2
  Constant1/1 -> Product1/2
  -S2(t)/1 -> Add2/2
  S1(t)/1 -> Add2/1
  Input Signal/1 -> Product1/1, Add/1
  Add2/1 -> DSBSC/1

== system signal_tranmission/SSB Demod33/Balanced Modulator1 ==
  note: -S2(t)
  note: S1(t)
  note: -m(t)
  note: m(t)
  note: S2(t)
  note: S1(t)
  Input Signal : Inport
  Carrier Signal : Inport  Port=2
  -S2(t) : Product
  Add : Sum
  Add1 : Sum
  Add2 : Sum
  Constant : Constant
  Constant1 : Constant  Value=-1
  Constant2 : Constant
  Constant3 : Constant  Value=-1
  Product1 : Product
  S1(t) : Product
  S2(t) : Product
  DSBSC : Outport
  wires:
  Product1/1 -> Add1/1
  Add/1 -> S1(t)/1
  Constant3/1 -> -S2(t)/2
  Constant2/1 -> Add1/2
  S2(t)/1 -> -S2(t)/1
  Carrier Signal/1 -> S1(t)/2, S2(t)/1
  Constant/1 -> Add/2
  Add1/1 -> S2(t)/2
  Constant1/1 -> Product1/2
  -S2(t)/1 -> Add2/2
  S1(t)/1 -> Add2/1
  Input Signal/1 -> Product1/1, Add/1
  Add2/1 -> DSBSC/1

== system signal_tranmission/SSB Demod34/Balanced Modulator1 ==
  note: -S2(t)
  note: S1(t)
  note: -m(t)
  note: m(t)
  note: S2(t)
  note: S1(t)
  Input Signal : Inport
  Carrier Signal : Inport  Port=2
  -S2(t) : Product
  Add : Sum
  Add1 : Sum
  Add2 : Sum
  Constant : Constant
  Constant1 : Constant  Value=-1
  Constant2 : Constant
  Constant3 : Constant  Value=-1
  Product1 : Product
  S1(t) : Product
  S2(t) : Product
  DSBSC : Outport
  wires:
  Product1/1 -> Add1/1
  Add/1 -> S1(t)/1
  Constant3/1 -> -S2(t)/2
  Constant2/1 -> Add1/2
  S2(t)/1 -> -S2(t)/1
  Carrier Signal/1 -> S1(t)/2, S2(t)/1
  Constant/1 -> Add/2
  Add1/1 -> S2(t)/2
  Constant1/1 -> Product1/2
  -S2(t)/1 -> Add2/2
  S1(t)/1 -> Add2/1
  Input Signal/1 -> Product1/1, Add/1
  Add2/1 -> DSBSC/1

== system signal_tranmission/SSB Demod35/Balanced Modulator1 ==
  note: -S2(t)
  note: S1(t)
  note: -m(t)
  note: m(t)
  note: S2(t)
  note: S1(t)
  Input Signal : Inport
  Carrier Signal : Inport  Port=2
  -S2(t) : Product
  Add : Sum
  Add1 : Sum
  Add2 : Sum
  Constant : Constant
  Constant1 : Constant  Value=-1
  Constant2 : Constant
  Constant3 : Constant  Value=-1
  Product1 : Product
  S1(t) : Product
  S2(t) : Product
  DSBSC : Outport
  wires:
  Product1/1 -> Add1/1
  Add/1 -> S1(t)/1
  Constant3/1 -> -S2(t)/2
  Constant2/1 -> Add1/2
  S2(t)/1 -> -S2(t)/1
  Carrier Signal/1 -> S1(t)/2, S2(t)/1
  Constant/1 -> Add/2
  Add1/1 -> S2(t)/2
  Constant1/1 -> Product1/2
  -S2(t)/1 -> Add2/2
  S1(t)/1 -> Add2/1
  Input Signal/1 -> Product1/1, Add/1
  Add2/1 -> DSBSC/1

== system signal_tranmission/SSB Demod36/Balanced Modulator1 ==
  note: -S2(t)
  note: S1(t)
  note: -m(t)
  note: m(t)
  note: S2(t)
  note: S1(t)
  Input Signal : Inport
  Carrier Signal : Inport  Port=2
  -S2(t) : Product
  Add : Sum
  Add1 : Sum
  Add2 : Sum
  Constant : Constant
  Constant1 : Constant  Value=-1
  Constant2 : Constant
  Constant3 : Constant  Value=-1
  Product1 : Product
  S1(t) : Product
  S2(t) : Product
  DSBSC : Outport
  wires:
  Product1/1 -> Add1/1
  Add/1 -> S1(t)/1
  Constant3/1 -> -S2(t)/2
  Constant2/1 -> Add1/2
  S2(t)/1 -> -S2(t)/1
  Carrier Signal/1 -> S1(t)/2, S2(t)/1
  Constant/1 -> Add/2
  Add1/1 -> S2(t)/2
  Constant1/1 -> Product1/2
  -S2(t)/1 -> Add2/2
  S1(t)/1 -> Add2/1
  Input Signal/1 -> Product1/1, Add/1
  Add2/1 -> DSBSC/1

== system signal_tranmission/SSB Demod37/Balanced Modulator1 ==
  note: -S2(t)
  note: S1(t)
  note: -m(t)
  note: m(t)
  note: S2(t)
  note: S1(t)
  Input Signal : Inport
  Carrier Signal : Inport  Port=2
  -S2(t) : Product
  Add : Sum
  Add1 : Sum
  Add2 : Sum
  Constant : Constant
  Constant1 : Constant  Value=-1
  Constant2 : Constant
  Constant3 : Constant  Value=-1
  Product1 : Product
  S1(t) : Product
  S2(t) : Product
  DSBSC : Outport
  wires:
  Product1/1 -> Add1/1
  Add/1 -> S1(t)/1
  Constant3/1 -> -S2(t)/2
  Constant2/1 -> Add1/2
  S2(t)/1 -> -S2(t)/1
  Carrier Signal/1 -> S1(t)/2, S2(t)/1
  Constant/1 -> Add/2
  Add1/1 -> S2(t)/2
  Constant1/1 -> Product1/2
  -S2(t)/1 -> Add2/2
  S1(t)/1 -> Add2/1
  Input Signal/1 -> Product1/1, Add/1
  Add2/1 -> DSBSC/1

== system signal_tranmission/SSB Demod38/Balanced Modulator1 ==
  note: -S2(t)
  note: S1(t)
  note: -m(t)
  note: m(t)
  note: S2(t)
  note: S1(t)
  Input Signal : Inport
  Carrier Signal : Inport  Port=2
  -S2(t) : Product
  Add : Sum
  Add1 : Sum
  Add2 : Sum
  Constant : Constant
  Constant1 : Constant  Value=-1
  Constant2 : Constant
  Constant3 : Constant  Value=-1
  Product1 : Product
  S1(t) : Product
  S2(t) : Product
  DSBSC : Outport
  wires:
  Product1/1 -> Add1/1
  Add/1 -> S1(t)/1
  Constant3/1 -> -S2(t)/2
  Constant2/1 -> Add1/2
  S2(t)/1 -> -S2(t)/1
  Carrier Signal/1 -> S1(t)/2, S2(t)/1
  Constant/1 -> Add/2
  Add1/1 -> S2(t)/2
  Constant1/1 -> Product1/2
  -S2(t)/1 -> Add2/2
  S1(t)/1 -> Add2/1
  Input Signal/1 -> Product1/1, Add/1
  Add2/1 -> DSBSC/1

== system signal_tranmission/SSB Demod39/Balanced Modulator1 ==
  note: -S2(t)
  note: S1(t)
  note: -m(t)
  note: m(t)
  note: S2(t)
  note: S1(t)
  Input Signal : Inport
  Carrier Signal : Inport  Port=2
  -S2(t) : Product
  Add : Sum
  Add1 : Sum
  Add2 : Sum
  Constant : Constant
  Constant1 : Constant  Value=-1
  Constant2 : Constant
  Constant3 : Constant  Value=-1
  Product1 : Product
  S1(t) : Product
  S2(t) : Product
  DSBSC : Outport
  wires:
  Product1/1 -> Add1/1
  Add/1 -> S1(t)/1
  Constant3/1 -> -S2(t)/2
  Constant2/1 -> Add1/2
  S2(t)/1 -> -S2(t)/1
  Carrier Signal/1 -> S1(t)/2, S2(t)/1
  Constant/1 -> Add/2
  Add1/1 -> S2(t)/2
  Constant1/1 -> Product1/2
  -S2(t)/1 -> Add2/2
  S1(t)/1 -> Add2/1
  Input Signal/1 -> Product1/1, Add/1
  Add2/1 -> DSBSC/1

== system signal_tranmission/SSB Demod4/Balanced Modulator1 ==
  note: -S2(t)
  note: S1(t)
  note: -m(t)
  note: m(t)
  note: S2(t)
  note: S1(t)
  Input Signal : Inport
  Carrier Signal : Inport  Port=2
  -S2(t) : Product
  Add : Sum
  Add1 : Sum
  Add2 : Sum
  Constant : Constant
  Constant1 : Constant  Value=-1
  Constant2 : Constant
  Constant3 : Constant  Value=-1
  Product1 : Product
  S1(t) : Product
  S2(t) : Product
  DSBSC : Outport
  wires:
  Product1/1 -> Add1/1
  Add/1 -> S1(t)/1
  Constant3/1 -> -S2(t)/2
  Constant2/1 -> Add1/2
  S2(t)/1 -> -S2(t)/1
  Carrier Signal/1 -> S1(t)/2, S2(t)/1
  Constant/1 -> Add/2
  Add1/1 -> S2(t)/2
  Constant1/1 -> Product1/2
  -S2(t)/1 -> Add2/2
  S1(t)/1 -> Add2/1
  Input Signal/1 -> Product1/1, Add/1
  Add2/1 -> DSBSC/1

== system signal_tranmission/SSB Demod40/Balanced Modulator1 ==
  note: -S2(t)
  note: S1(t)
  note: -m(t)
  note: m(t)
  note: S2(t)
  note: S1(t)
  Input Signal : Inport
  Carrier Signal : Inport  Port=2
  -S2(t) : Product
  Add : Sum
  Add1 : Sum
  Add2 : Sum
  Constant : Constant
  Constant1 : Constant  Value=-1
  Constant2 : Constant
  Constant3 : Constant  Value=-1
  Product1 : Product
  S1(t) : Product
  S2(t) : Product
  DSBSC : Outport
  wires:
  Product1/1 -> Add1/1
  Add/1 -> S1(t)/1
  Constant3/1 -> -S2(t)/2
  Constant2/1 -> Add1/2
  S2(t)/1 -> -S2(t)/1
  Carrier Signal/1 -> S1(t)/2, S2(t)/1
  Constant/1 -> Add/2
  Add1/1 -> S2(t)/2
  Constant1/1 -> Product1/2
  -S2(t)/1 -> Add2/2
  S1(t)/1 -> Add2/1
  Input Signal/1 -> Product1/1, Add/1
  Add2/1 -> DSBSC/1

== system signal_tranmission/SSB Demod41/Balanced Modulator1 ==
  note: -S2(t)
  note: S1(t)
  note: -m(t)
  note: m(t)
  note: S2(t)
  note: S1(t)
  Input Signal : Inport
  Carrier Signal : Inport  Port=2
  -S2(t) : Product
  Add : Sum
  Add1 : Sum
  Add2 : Sum
  Constant : Constant
  Constant1 : Constant  Value=-1
  Constant2 : Constant
  Constant3 : Constant  Value=-1
  Product1 : Product
  S1(t) : Product
  S2(t) : Product
  DSBSC : Outport
  wires:
  Product1/1 -> Add1/1
  Add/1 -> S1(t)/1
  Constant3/1 -> -S2(t)/2
  Constant2/1 -> Add1/2
  S2(t)/1 -> -S2(t)/1
  Carrier Signal/1 -> S1(t)/2, S2(t)/1
  Constant/1 -> Add/2
  Add1/1 -> S2(t)/2
  Constant1/1 -> Product1/2
  -S2(t)/1 -> Add2/2
  S1(t)/1 -> Add2/1
  Input Signal/1 -> Product1/1, Add/1
  Add2/1 -> DSBSC/1

== system signal_tranmission/SSB Demod42/Balanced Modulator1 ==
  note: -S2(t)
  note: S1(t)
  note: -m(t)
  note: m(t)
  note: S2(t)
  note: S1(t)
  Input Signal : Inport
  Carrier Signal : Inport  Port=2
  -S2(t) : Product
  Add : Sum
  Add1 : Sum
  Add2 : Sum
  Constant : Constant
  Constant1 : Constant  Value=-1
  Constant2 : Constant
  Constant3 : Constant  Value=-1
  Product1 : Product
  S1(t) : Product
  S2(t) : Product
  DSBSC : Outport
  wires:
  Product1/1 -> Add1/1
  Add/1 -> S1(t)/1
  Constant3/1 -> -S2(t)/2
  Constant2/1 -> Add1/2
  S2(t)/1 -> -S2(t)/1
  Carrier Signal/1 -> S1(t)/2, S2(t)/1
  Constant/1 -> Add/2
  Add1/1 -> S2(t)/2
  Constant1/1 -> Product1/2
  -S2(t)/1 -> Add2/2
  S1(t)/1 -> Add2/1
  Input Signal/1 -> Product1/1, Add/1
  Add2/1 -> DSBSC/1

== system signal_tranmission/SSB Demod43/Balanced Modulator1 ==
  note: -S2(t)
  note: S1(t)
  note: -m(t)
  note: m(t)
  note: S2(t)
  note: S1(t)
  Input Signal : Inport
  Carrier Signal : Inport  Port=2
  -S2(t) : Product
  Add : Sum
  Add1 : Sum
  Add2 : Sum
  Constant : Constant
  Constant1 : Constant  Value=-1
  Constant2 : Constant
  Constant3 : Constant  Value=-1
  Product1 : Product
  S1(t) : Product
  S2(t) : Product
  DSBSC : Outport
  wires:
  Product1/1 -> Add1/1
  Add/1 -> S1(t)/1
  Constant3/1 -> -S2(t)/2
  Constant2/1 -> Add1/2
  S2(t)/1 -> -S2(t)/1
  Carrier Signal/1 -> S1(t)/2, S2(t)/1
  Constant/1 -> Add/2
  Add1/1 -> S2(t)/2
  Constant1/1 -> Product1/2
  -S2(t)/1 -> Add2/2
  S1(t)/1 -> Add2/1
  Input Signal/1 -> Product1/1, Add/1
  Add2/1 -> DSBSC/1

== system signal_tranmission/SSB Demod44/Balanced Modulator1 ==
  note: -S2(t)
  note: S1(t)
  note: -m(t)
  note: m(t)
  note: S2(t)
  note: S1(t)
  Input Signal : Inport
  Carrier Signal : Inport  Port=2
  -S2(t) : Product
  Add : Sum
  Add1 : Sum
  Add2 : Sum
  Constant : Constant
  Constant1 : Constant  Value=-1
  Constant2 : Constant
  Constant3 : Constant  Value=-1
  Product1 : Product
  S1(t) : Product
  S2(t) : Product
  DSBSC : Outport
  wires:
  Product1/1 -> Add1/1
  Add/1 -> S1(t)/1
  Constant3/1 -> -S2(t)/2
  Constant2/1 -> Add1/2
  S2(t)/1 -> -S2(t)/1
  Carrier Signal/1 -> S1(t)/2, S2(t)/1
  Constant/1 -> Add/2
  Add1/1 -> S2(t)/2
  Constant1/1 -> Product1/2
  -S2(t)/1 -> Add2/2
  S1(t)/1 -> Add2/1
  Input Signal/1 -> Product1/1, Add/1
  Add2/1 -> DSBSC/1

== system signal_tranmission/SSB Demod45/Balanced Modulator1 ==
  note: -S2(t)
  note: S1(t)
  note: -m(t)
  note: m(t)
  note: S2(t)
  note: S1(t)
  Input Signal : Inport
  Carrier Signal : Inport  Port=2
  -S2(t) : Product
  Add : Sum
  Add1 : Sum
  Add2 : Sum
  Constant : Constant
  Constant1 : Constant  Value=-1
  Constant2 : Constant
  Constant3 : Constant  Value=-1
  Product1 : Product
  S1(t) : Product
  S2(t) : Product
  DSBSC : Outport
  wires:
  Product1/1 -> Add1/1
  Add/1 -> S1(t)/1
  Constant3/1 -> -S2(t)/2
  Constant2/1 -> Add1/2
  S2(t)/1 -> -S2(t)/1
  Carrier Signal/1 -> S1(t)/2, S2(t)/1
  Constant/1 -> Add/2
  Add1/1 -> S2(t)/2
  Constant1/1 -> Product1/2
  -S2(t)/1 -> Add2/2
  S1(t)/1 -> Add2/1
  Input Signal/1 -> Product1/1, Add/1
  Add2/1 -> DSBSC/1

== system signal_tranmission/SSB Demod46/Balanced Modulator1 ==
  note: -S2(t)
  note: S1(t)
  note: -m(t)
  note: m(t)
  note: S2(t)
  note: S1(t)
  Input Signal : Inport
  Carrier Signal : Inport  Port=2
  -S2(t) : Product
  Add : Sum
  Add1 : Sum
  Add2 : Sum
  Constant : Constant
  Constant1 : Constant  Value=-1
  Constant2 : Constant
  Constant3 : Constant  Value=-1
  Product1 : Product
  S1(t) : Product
  S2(t) : Product
  DSBSC : Outport
  wires:
  Product1/1 -> Add1/1
  Add/1 -> S1(t)/1
  Constant3/1 -> -S2(t)/2
  Constant2/1 -> Add1/2
  S2(t)/1 -> -S2(t)/1
  Carrier Signal/1 -> S1(t)/2, S2(t)/1
  Constant/1 -> Add/2
  Add1/1 -> S2(t)/2
  Constant1/1 -> Product1/2
  -S2(t)/1 -> Add2/2
  S1(t)/1 -> Add2/1
  Input Signal/1 -> Product1/1, Add/1
  Add2/1 -> DSBSC/1

== system signal_tranmission/SSB Demod47/Balanced Modulator1 ==
  note: -S2(t)
  note: S1(t)
  note: -m(t)
  note: m(t)
  note: S2(t)
  note: S1(t)
  Input Signal : Inport
  Carrier Signal : Inport  Port=2
  -S2(t) : Product
  Add : Sum
  Add1 : Sum
  Add2 : Sum
  Constant : Constant
  Constant1 : Constant  Value=-1
  Constant2 : Constant
  Constant3 : Constant  Value=-1
  Product1 : Product
  S1(t) : Product
  S2(t) : Product
  DSBSC : Outport
  wires:
  Product1/1 -> Add1/1
  Add/1 -> S1(t)/1
  Constant3/1 -> -S2(t)/2
  Constant2/1 -> Add1/2
  S2(t)/1 -> -S2(t)/1
  Carrier Signal/1 -> S1(t)/2, S2(t)/1
  Constant/1 -> Add/2
  Add1/1 -> S2(t)/2
  Constant1/1 -> Product1/2
  -S2(t)/1 -> Add2/2
  S1(t)/1 -> Add2/1
  Input Signal/1 -> Product1/1, Add/1
  Add2/1 -> DSBSC/1

== system signal_tranmission/SSB Demod48/Balanced Modulator1 ==
  note: -S2(t)
  note: S1(t)
  note: -m(t)
  note: m(t)
  note: S2(t)
  note: S1(t)
  Input Signal : Inport
  Carrier Signal : Inport  Port=2
  -S2(t) : Product
  Add : Sum
  Add1 : Sum
  Add2 : Sum
  Constant : Constant
  Constant1 : Constant  Value=-1
  Constant2 : Constant
  Constant3 : Constant  Value=-1
  Product1 : Product
  S1(t) : Product
  S2(t) : Product
  DSBSC : Outport
  wires:
  Product1/1 -> Add1/1
  Add/1 -> S1(t)/1
  Constant3/1 -> -S2(t)/2
  Constant2/1 -> Add1/2
  S2(t)/1 -> -S2(t)/1
  Carrier Signal/1 -> S1(t)/2, S2(t)/1
  Constant/1 -> Add/2
  Add1/1 -> S2(t)/2
  Constant1/1 -> Product1/2
  -S2(t)/1 -> Add2/2
  S1(t)/1 -> Add2/1
  Input Signal/1 -> Product1/1, Add/1
  Add2/1 -> DSBSC/1

== system signal_tranmission/SSB Demod49/Balanced Modulator1 ==
  note: -S2(t)
  note: S1(t)
  note: -m(t)
  note: m(t)
  note: S2(t)
  note: S1(t)
  Input Signal : Inport
  Carrier Signal : Inport  Port=2
  -S2(t) : Product
  Add : Sum
  Add1 : Sum
  Add2 : Sum
  Constant : Constant
  Constant1 : Constant  Value=-1
  Constant2 : Constant
  Constant3 : Constant  Value=-1
  Product1 : Product
  S1(t) : Product
  S2(t) : Product
  DSBSC : Outport
  wires:
  Product1/1 -> Add1/1
  Add/1 -> S1(t)/1
  Constant3/1 -> -S2(t)/2
  Constant2/1 -> Add1/2
  S2(t)/1 -> -S2(t)/1
  Carrier Signal/1 -> S1(t)/2, S2(t)/1
  Constant/1 -> Add/2
  Add1/1 -> S2(t)/2
  Constant1/1 -> Product1/2
  -S2(t)/1 -> Add2/2
  S1(t)/1 -> Add2/1
  Input Signal/1 -> Product1/1, Add/1
  Add2/1 -> DSBSC/1

== system signal_tranmission/SSB Demod5/Balanced Modulator1 ==
  note: -S2(t)
  note: S1(t)
  note: -m(t)
  note: m(t)
  note: S2(t)
  note: S1(t)
  Input Signal : Inport
  Carrier Signal : Inport  Port=2
  -S2(t) : Product
  Add : Sum
  Add1 : Sum
  Add2 : Sum
  Constant : Constant
  Constant1 : Constant  Value=-1
  Constant2 : Constant
  Constant3 : Constant  Value=-1
  Product1 : Product
  S1(t) : Product
  S2(t) : Product
  DSBSC : Outport
  wires:
  Product1/1 -> Add1/1
  Add/1 -> S1(t)/1
  Constant3/1 -> -S2(t)/2
  Constant2/1 -> Add1/2
  S2(t)/1 -> -S2(t)/1
  Carrier Signal/1 -> S1(t)/2, S2(t)/1
  Constant/1 -> Add/2
  Add1/1 -> S2(t)/2
  Constant1/1 -> Product1/2
  -S2(t)/1 -> Add2/2
  S1(t)/1 -> Add2/1
  Input Signal/1 -> Product1/1, Add/1
  Add2/1 -> DSBSC/1

== system signal_tranmission/SSB Demod50/Balanced Modulator1 ==
  note: -S2(t)
  note: S1(t)
  note: -m(t)
  note: m(t)
  note: S2(t)
  note: S1(t)
  Input Signal : Inport
  Carrier Signal : Inport  Port=2
  -S2(t) : Product
  Add : Sum
  Add1 : Sum
  Add2 : Sum
  Constant : Constant
  Constant1 : Constant  Value=-1
  Constant2 : Constant
  Constant3 : Constant  Value=-1
  Product1 : Product
  S1(t) : Product
  S2(t) : Product
  DSBSC : Outport
  wires:
  Product1/1 -> Add1/1
  Add/1 -> S1(t)/1
  Constant3/1 -> -S2(t)/2
  Constant2/1 -> Add1/2
  S2(t)/1 -> -S2(t)/1
  Carrier Signal/1 -> S1(t)/2, S2(t)/1
  Constant/1 -> Add/2
  Add1/1 -> S2(t)/2
  Constant1/1 -> Product1/2
  -S2(t)/1 -> Add2/2
  S1(t)/1 -> Add2/1
  Input Signal/1 -> Product1/1, Add/1
  Add2/1 -> DSBSC/1

== system signal_tranmission/SSB Demod51/Balanced Modulator1 ==
  note: -S2(t)
  note: S1(t)
  note: -m(t)
  note: m(t)
  note: S2(t)
  note: S1(t)
  Input Signal : Inport
  Carrier Signal : Inport  Port=2
  -S2(t) : Product
  Add : Sum
  Add1 : Sum
  Add2 : Sum
  Constant : Constant
  Constant1 : Constant  Value=-1
  Constant2 : Constant
  Constant3 : Constant  Value=-1
  Product1 : Product
  S1(t) : Product
  S2(t) : Product
  DSBSC : Outport
  wires:
  Product1/1 -> Add1/1
  Add/1 -> S1(t)/1
  Constant3/1 -> -S2(t)/2
  Constant2/1 -> Add1/2
  S2(t)/1 -> -S2(t)/1
  Carrier Signal/1 -> S1(t)/2, S2(t)/1
  Constant/1 -> Add/2
  Add1/1 -> S2(t)/2
  Constant1/1 -> Product1/2
  -S2(t)/1 -> Add2/2
  S1(t)/1 -> Add2/1
  Input Signal/1 -> Product1/1, Add/1
  Add2/1 -> DSBSC/1

== system signal_tranmission/SSB Demod52/Balanced Modulator1 ==
  note: -S2(t)
  note: S1(t)
  note: -m(t)
  note: m(t)
  note: S2(t)
  note: S1(t)
  Input Signal : Inport
  Carrier Signal : Inport  Port=2
  -S2(t) : Product
  Add : Sum
  Add1 : Sum
  Add2 : Sum
  Constant : Constant
  Constant1 : Constant  Value=-1
  Constant2 : Constant
  Constant3 : Constant  Value=-1
  Product1 : Product
  S1(t) : Product
  S2(t) : Product
  DSBSC : Outport
  wires:
  Product1/1 -> Add1/1
  Add/1 -> S1(t)/1
  Constant3/1 -> -S2(t)/2
  Constant2/1 -> Add1/2
  S2(t)/1 -> -S2(t)/1
  Carrier Signal/1 -> S1(t)/2, S2(t)/1
  Constant/1 -> Add/2
  Add1/1 -> S2(t)/2
  Constant1/1 -> Product1/2
  -S2(t)/1 -> Add2/2
  S1(t)/1 -> Add2/1
  Input Signal/1 -> Product1/1, Add/1
  Add2/1 -> DSBSC/1

== system signal_tranmission/SSB Demod53/Balanced Modulator1 ==
  note: -S2(t)
  note: S1(t)
  note: -m(t)
  note: m(t)
  note: S2(t)
  note: S1(t)
  Input Signal : Inport
  Carrier Signal : Inport  Port=2
  -S2(t) : Product
  Add : Sum
  Add1 : Sum
  Add2 : Sum
  Constant : Constant
  Constant1 : Constant  Value=-1
  Constant2 : Constant
  Constant3 : Constant  Value=-1
  Product1 : Product
  S1(t) : Product
  S2(t) : Product
  DSBSC : Outport
  wires:
  Product1/1 -> Add1/1
  Add/1 -> S1(t)/1
  Constant3/1 -> -S2(t)/2
  Constant2/1 -> Add1/2
  S2(t)/1 -> -S2(t)/1
  Carrier Signal/1 -> S1(t)/2, S2(t)/1
  Constant/1 -> Add/2
  Add1/1 -> S2(t)/2
  Constant1/1 -> Product1/2
  -S2(t)/1 -> Add2/2
  S1(t)/1 -> Add2/1
  Input Signal/1 -> Product1/1, Add/1
  Add2/1 -> DSBSC/1

== system signal_tranmission/SSB Demod54/Balanced Modulator1 ==
  note: -S2(t)
  note: S1(t)
  note: -m(t)
  note: m(t)
  note: S2(t)
  note: S1(t)
  Input Signal : Inport
  Carrier Signal : Inport  Port=2
  -S2(t) : Product
  Add : Sum
  Add1 : Sum
  Add2 : Sum
  Constant : Constant
  Constant1 : Constant  Value=-1
  Constant2 : Constant
  Constant3 : Constant  Value=-1
  Product1 : Product
  S1(t) : Product
  S2(t) : Product
  DSBSC : Outport
  wires:
  Product1/1 -> Add1/1
  Add/1 -> S1(t)/1
  Constant3/1 -> -S2(t)/2
  Constant2/1 -> Add1/2
  S2(t)/1 -> -S2(t)/1
  Carrier Signal/1 -> S1(t)/2, S2(t)/1
  Constant/1 -> Add/2
  Add1/1 -> S2(t)/2
  Constant1/1 -> Product1/2
  -S2(t)/1 -> Add2/2
  S1(t)/1 -> Add2/1
  Input Signal/1 -> Product1/1, Add/1
  Add2/1 -> DSBSC/1
